simulink model "LDM_closed_loop"  (R2019b)
settings: Solver=FixedStepDiscrete  StartTime=0.0  StopTime=inf  FixedStep=0.01  RelTol=1e-3  EnableMultiTasking=on
settings Model: PauseTimes=341.0  Creator=btc2abt  LastModifiedBy=DOT1BP
settings DataIOCC: LimitDataPoints=on  ReturnWorkspaceOutputs=off
settings OptimizationCC: LifeSpan=inf
settings DebuggingCC: MultiTaskRateTransMsg=warning  AllowSymbolicDim=off  SFUnexpectedBacktrackingDiag=warning  SFNoUnconditionalDefaultTransitionDiag=warning  SFExecutionAtInitializationDiag=none  ArithmeticOperatorsInVariantConditions=warning
settings ModelReferenceCC: ModelReferenceNumInstancesAllowed=Single  PropagateSignalLabelsOutOfModel=off
settings SFSimCC: SimUseLocalCustomCode=off  CustomCodeUndefinedFunction=UseInterfaceOnly
settings RTWCC: RTWUseLocalCustomCode=off
settings CodeAppCC: StateflowObjectComments=on
settings GRTTargetCC: TargetLangStandard=C89/C90 (ANSI)
settings ConfigComp: CovMetricSettings=dw  CovHtmlReporting=on  CovSaveCumulativeToWorkspaceVar=on  CovSaveSingleToWorkspaceVar=on  CovExternalEMLEnable=off

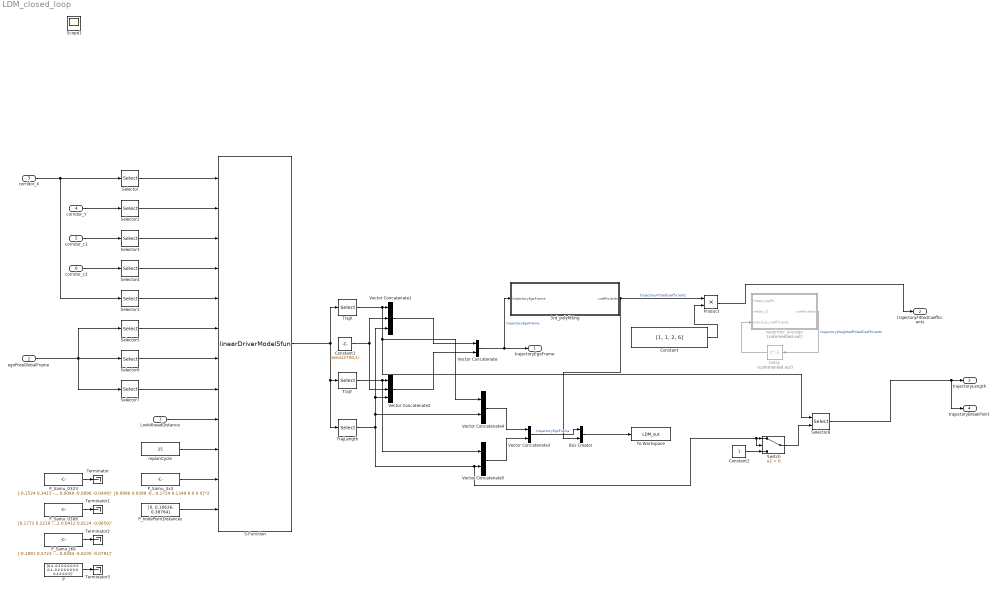
== system LDM_closed_loop ==
  LookAheadDistance : Inport
  egoPoseGlobalFrame : Inport  Port=2
  corridor_X : Inport  Port=3
  corridor_Y : Inport  Port=4
  corridor_c1 : Inport  Port=5
  corridor_c2 : Inport  Port=6
  3rd_polyfitting : MATLAB Function  TreatAsAtomicUnit=on
  Bus Creator : BusCreator  Inputs=2
  Constant : Constant  Value=[1, 1, 2, 6]
  Constant1 : Constant  Value=zeros(2700,1)
  Constant2 : Constant
  Delay : Delay  Commented=on  DelayLength=1
  P : Constant  Value=[0.4 -0.2 0 0 0 0 0 0 0.4 -0.2 0 0 0 0 0 0 0.4 0 0 0 0]'
  P_Samu_0308 : Constant  Value=[0.1773 0.2219 -0.2682 -0.0332 0.0887 0.0013 0.0761 -0.3368 0.7714 -0.3123 0.0194 -0.0027 0.0293 0.0384 0.2913 -0.4504 0.2953 -0.0362 0.0412 0.0124 -0.0650]'
  P_Samu_0323 : Constant  Value=[-0.1524 0.3415 -0.1253 -0.0464 0.0239 -0.0055 0.0215 0.1143 0.0686 -0.1218 -0.0161 0.0354 0.0297 -0.0039 0.3901 -0.5318 0.2184 0.0146 0.0089 -0.0096 -0.0449]'
  P_Samu_3x3 : Constant  Value=[0.0996 0.0399 -0.0811 0 0 0 0 -0.0754 0.2313 -0.0940 0 0 0 0 0.1228 -0.1724 0.1349 0 0 0 0]'*2
  P_Samu_JKK : Constant  Value=[-0.1891 0.5723 -0.2526 -0.0105 0.0167 -0.0250 0.0681 -0.4980 0.9711 -0.3461 0.0010 -0.0047 0.0333 0.0391 0.6295 -0.8867 0.3919 0.0183 0.0494 -0.0235 -0.0791]'
  P_nodePointDistances : Constant  Value=[0, 0.10636, 0.38764]
  Product : Product
  S-Function : S-Function  FunctionName=linearDriverModelSfun  SFunctionDeploymentMode=off  EnableBusSupport=off
  Selector{,2..4} (4 alike) : Selector  InputPortWidth=301  IndexOptions=Index vector (dialog)  Indices=linspace(1,300,300)  OutputSizes=1
  Selector1 : Selector  InputPortWidth=301  IndexOptions=Index vector (dialog)  Indices=301  OutputSizes=1
  Selector5 : Selector  InputPortWidth=3  IndexOptions=Index vector (dialog)  Indices=1  OutputSizes=1
  Selector6 : Selector  InputPortWidth=3  IndexOptions=Index vector (dialog)  Indices=2  OutputSizes=1
  Selector7 : Selector  InputPortWidth=3  IndexOptions=Index vector (dialog)  Indices=3  OutputSizes=1
  Selector8 : Selector  InputPortWidth=300  IndexOptions=Index vector (port)  Indices=[1 3]  OutputSizes=1
  Switch : Switch  Criteria=u2 > Threshold
  Terminator{,1..3} (4 alike) : Terminator
  To Workspace : ToWorkspace  VariableName=LDM_out  SaveFormat=Timeseries  SampleTime=-1
  TrajLength : Selector  InputPortWidth=601  IndexOptions=Index vector (dialog)  Indices=601  OutputSizes=1
  TrajX : Selector  InputPortWidth=601  IndexOptions=Index vector (dialog)  Indices=linspace(1,300,300)  OutputSizes=1
  TrajY : Selector  InputPortWidth=601  IndexOptions=Index vector (dialog)  Indices=linspace(301,600,300)  OutputSizes=1
  Vector Concatenate : Concatenate  Mode=Multidimensional array  ConcatenateDimension=2
  Vector Concatenate1 : Concatenate  NumInputs=3
  Vector Concatenate2 : Concatenate  NumInputs=3
  Vector Concatenate3 : Concatenate  Mode=Multidimensional array  ConcatenateDimension=2
  Vector Concatenate4 : Concatenate
  Vector Concatenate5 : Concatenate
  replanCycle : Constant  Value=25
  weighted_average : MATLAB Function  Commented=on  TreatAsAtomicUnit=on
  trajectoryEgoFrame : Outport
  trajectoryFittedCoefficients : Outport  Port=2
  trajectoryLength : Outport  Port=3
  trajectoryBreakPoint : Outport  Port=4
  Scope1 : Scope
  wires:
  P_Samu_3x3/1 -> S-Function/11
  P_nodePointDistances/1 -> S-Function/12
  replanCycle/1 -> S-Function/10
  S-Function/1 -> TrajY/1, TrajLength/1, TrajX/1
  Selector/1 -> S-Function/1
  Selector2/1 -> S-Function/2
  Selector3/1 -> S-Function/3
  Selector4/1 -> S-Function/4
  corridor_X/1 -> Selector/1, Selector1/1
  Selector1/1 -> S-Function/5
  corridor_c2/1 -> Selector4/1
  corridor_c1/1 -> Selector3/1
  corridor_Y/1 -> Selector2/1
  LookAheadDistance/1 -> S-Function/9
  egoPoseGlobalFrame/1 -> Selector7/1, Selector6/1, Selector5/1
  Selector5/1 -> S-Function/6
  Selector6/1 -> S-Function/7
  Selector7/1 -> S-Function/8
  Vector Concatenate/1 -> 3rd_polyfitting/1(trajectoryEgoFrame), trajectoryEgoFrame/1  "trajectoryEgoFrame"
  Constant1/1 -> Vector Concatenate2/2, Vector Concatenate1/2
  TrajX/1 -> Vector Concatenate4/1, Selector8/1, Vector Concatenate1/1
  TrajLength/1 -> Vector Concatenate2/3, Vector Concatenate1/3, Vector Concatenate4/2, Switch/2, Switch/1, Vector Concatenate5/2
  TrajY/1 -> Vector Concatenate5/1, Vector Concatenate2/1
  Vector Concatenate2/1 -> Vector Concatenate/2
  Vector Concatenate1/1 -> Vector Concatenate/1
  P_Samu_0323/1 -> Terminator/1
  P_Samu_0308/1 -> Terminator1/1
  P_Samu_JKK/1 -> Terminator2/1
  Vector Concatenate3/1 -> Bus Creator/1  "trajectoryEgoFrame"
  Vector Concatenate4/1 -> Vector Concatenate3/1
  Vector Concatenate5/1 -> Vector Concatenate3/2
  Bus Creator/1 -> To Workspace/1
  3rd_polyfitting/1(coefficients) -> Product/1, Bus Creator/2  "trajectoryFittedCoefficients"
  Constant/1 -> Product/2
  weighted_average/1(coefficients) -> Delay/1  "trajectoryWeightedFittedCoefficients"
  Product/1 -> trajectoryFittedCoefficients/1
  Delay/1 -> weighted_average/3(previous_coefficients)
  Switch/1 -> Selector8/2
  Constant2/1 -> Switch/3
  Selector8/1 -> trajectoryBreakPoint/1, trajectoryLength/1
  P/1 -> Terminator3/1

== matlab function LDM_closed_loop/weighted_average ==
  data: fitted_coeffs input; coefficients output; reflat_c2 input; previous_coefficients input
function coefficients  = fcn(fitted_coeffs, reflat_c2, previous_coefficients)

coefficients = fitted_coeffs;
c = 0.03;

currentC3 = abs(coefficients(4));
x_LUT = [0 1e-7 5e-6 1e-5 3e-5 6e-5 1e-4];
weights = [1 1 0.7 0.4 0.2 0.1 0];

weight = interp1(x_LUT, weights, currentC3);

coefficients(3) = (coefficients(3) * weight) + (reflat_c2 * (1 - weight));
coefficients(3) = previous_coefficients(3)*(1-c)+coefficients(3)*c;

end

== matlab function LDM_closed_loop/3rd_polyfitting ==
  data: trajectoryEgoFrame input; coefficients output
function coefficients  = fitPoly3rdOrder(trajectoryEgoFrame)

n = trajectoryEgoFrame(3001,1);

%reduced_traj = reducepoly(trajectoryEgoFrame(1:n,:), 0.0005);
if n > 0
    p = polyfit(trajectoryEgoFrame(1:n,1), trajectoryEgoFrame(1:n,2), 3);
    coefficients = [p(4) p(3) p(2) p(1)];
else
    coefficients = [0 0 0 0];
end

end
